simulink model "Trigger_Subsystem"  (R2024b)
settings: Solver=FixedStepAuto  StartTime=0.0  StopTime=8  FixedStep=0.001  RelTol=1e-3
settings Model: Creator=abdal  LastModifiedBy=abdal

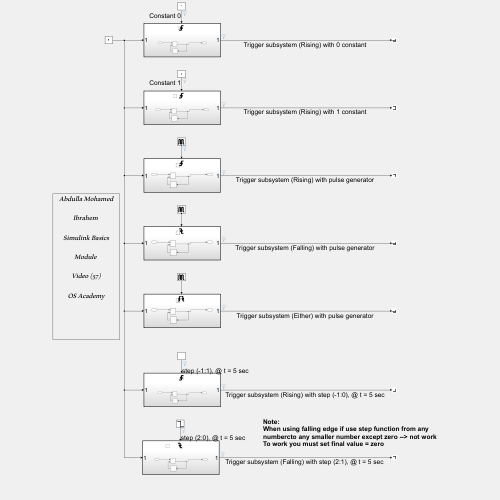
[thumbnail: Simulink's stored preview of the top-level diagram]
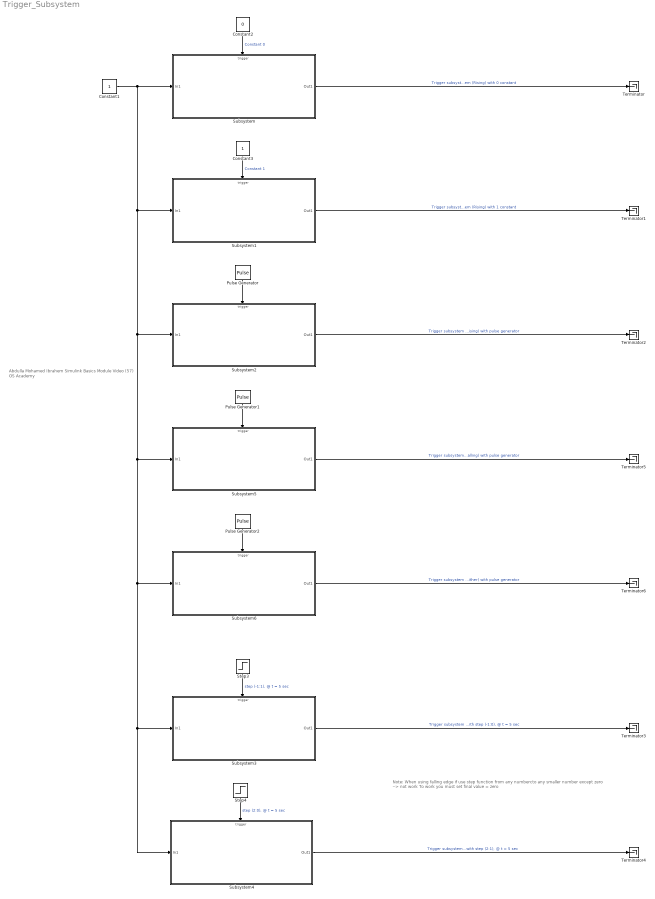
== system Trigger_Subsystem ==
  note: Note:
      | When using falling edge if use step function from any numbercto any smaller number except zero --> not work
      | To work you must set final value = zero
  note: Abdulla Mohamed Ibrahem
      | Simulink Basics Module
      | Video (57)
      | OS Academy
  Constant1 : Constant
  Constant2 : Constant  Value=0
  Constant3 : Constant
  Pulse Generator : DiscretePulseGenerator  PulseType=Time based  PulseWidth=50
  Pulse Generator1 : DiscretePulseGenerator  PulseType=Time based  PulseWidth=50
  Pulse Generator2 : DiscretePulseGenerator  PulseType=Time based  PulseWidth=50
  Step3 : Step  Time=5  Before=-1  After=0  SampleTime=0
  Step4 : Step  Time=5  Before=2  After=0  SampleTime=0
  Subsystem : Subsystem  TreatAsAtomicUnit=on
  Subsystem1 : Subsystem  TreatAsAtomicUnit=on
  Subsystem2 : Subsystem  TreatAsAtomicUnit=on
  Subsystem3 : Subsystem  TreatAsAtomicUnit=on
  Subsystem4 : Subsystem  TreatAsAtomicUnit=on
  Subsystem5 : Subsystem  TreatAsAtomicUnit=on
  Subsystem6 : Subsystem  TreatAsAtomicUnit=on
  Terminator{,1..6} (7 alike) : Terminator
  wires:
  Subsystem4/1(Out1) -> Terminator4/1  "Trigger subsystem (Falling) with step (2:1), @ t = 5 sec"
  Constant1/1 -> Subsystem/1(In1), Subsystem5/1(In1), Subsystem6/1(In1), Subsystem4/1(In1), Subsystem3/1(In1), Subsystem2/1(In1), Subsystem1/1(In1)
  Step4/1 -> Subsystem4/Trigger  "step (2:0), @ t = 5 sec"
  Subsystem/1(Out1) -> Terminator/1  "Trigger subsystem (Rising) with 0 constant"
  Step3/1 -> Subsystem3/Trigger  "step (-1:1), @ t = 5 sec"
  Subsystem1/1(Out1) -> Terminator1/1  "Trigger subsystem (Rising) with 1 constant"
  Subsystem2/1(Out1) -> Terminator2/1  "Trigger subsystem (Rising) with pulse generator"
  Subsystem3/1(Out1) -> Terminator3/1  "Trigger subsystem (Rising) with step (-1:0), @ t = 5 sec"
  Constant2/1 -> Subsystem/Trigger  "Constant 0"
  Constant3/1 -> Subsystem1/Trigger  "Constant 1"
  Pulse Generator/1 -> Subsystem2/Trigger
  Pulse Generator1/1 -> Subsystem5/Trigger
  Subsystem5/1(Out1) -> Terminator5/1  "Trigger subsystem (Falling) with pulse generator"
  Subsystem6/1(Out1) -> Terminator6/1  "Trigger subsystem (Either) with pulse generator"
  Pulse Generator2/1 -> Subsystem6/Trigger

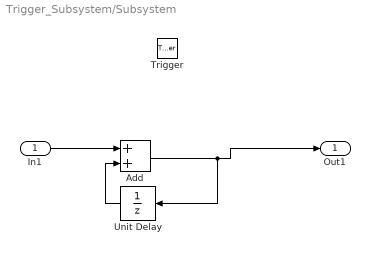
== system Trigger_Subsystem/Subsystem ==
  In1 : Inport
  Trigger : TriggerPort  VariantControl=(inherit)  PortDimensions=1
  Add : Sum
  Unit Delay : UnitDelay  SampleTime=-1  HasFrameUpgradeWarning=on
  Out1 : Outport
  wires:
  In1/1 -> Add/1
  Add/1 -> Unit Delay/1, Out1/1
  Unit Delay/1 -> Add/2

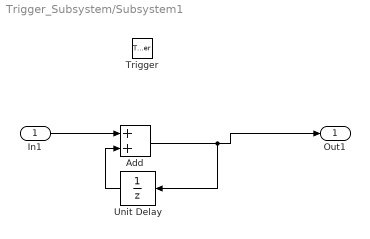
== system Trigger_Subsystem/Subsystem1 ==
  In1 : Inport
  Trigger : TriggerPort  VariantControl=(inherit)  PortDimensions=1
  Add : Sum
  Unit Delay : UnitDelay  SampleTime=-1  HasFrameUpgradeWarning=on
  Out1 : Outport
  wires:
  Unit Delay/1 -> Add/2
  Add/1 -> Out1/1, Unit Delay/1
  In1/1 -> Add/1

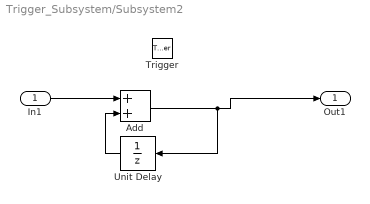
== system Trigger_Subsystem/Subsystem2 ==
  In1 : Inport
  Trigger : TriggerPort  VariantControl=(inherit)  PortDimensions=1
  Add : Sum
  Unit Delay : UnitDelay  SampleTime=-1  HasFrameUpgradeWarning=on
  Out1 : Outport
  wires:
  In1/1 -> Add/1
  Add/1 -> Unit Delay/1, Out1/1
  Unit Delay/1 -> Add/2

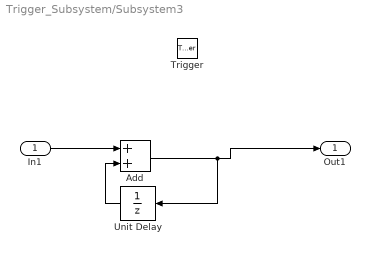
== system Trigger_Subsystem/Subsystem3 ==
  In1 : Inport
  Trigger : TriggerPort  VariantControl=(inherit)  PortDimensions=1
  Add : Sum
  Unit Delay : UnitDelay  SampleTime=-1  HasFrameUpgradeWarning=on
  Out1 : Outport
  wires:
  Unit Delay/1 -> Add/2
  Add/1 -> Out1/1, Unit Delay/1
  In1/1 -> Add/1

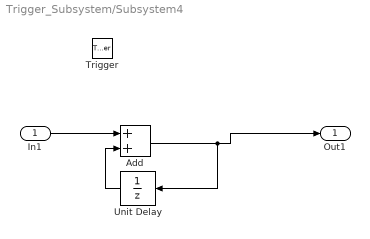
== system Trigger_Subsystem/Subsystem4 ==
  In1 : Inport
  Trigger : TriggerPort  TriggerType=falling  VariantControl=(inherit)  PortDimensions=1
  Add : Sum
  Unit Delay : UnitDelay  SampleTime=-1  HasFrameUpgradeWarning=on
  Out1 : Outport
  wires:
  In1/1 -> Add/1
  Add/1 -> Unit Delay/1, Out1/1
  Unit Delay/1 -> Add/2

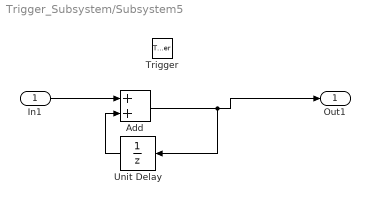
== system Trigger_Subsystem/Subsystem5 ==
  In1 : Inport
  Trigger : TriggerPort  TriggerType=falling  VariantControl=(inherit)  PortDimensions=1
  Add : Sum
  Unit Delay : UnitDelay  SampleTime=-1  HasFrameUpgradeWarning=on
  Out1 : Outport
  wires:
  Unit Delay/1 -> Add/2
  Add/1 -> Out1/1, Unit Delay/1
  In1/1 -> Add/1

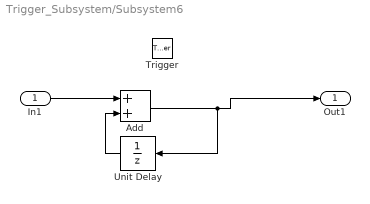
== system Trigger_Subsystem/Subsystem6 ==
  In1 : Inport
  Trigger : TriggerPort  TriggerType=either  VariantControl=(inherit)  PortDimensions=1
  Add : Sum
  Unit Delay : UnitDelay  SampleTime=-1  HasFrameUpgradeWarning=on
  Out1 : Outport
  wires:
  In1/1 -> Add/1
  Add/1 -> Unit Delay/1, Out1/1
  Unit Delay/1 -> Add/2
